simulink model "sstv_receive"  (R2022a)
settings: Solver=FixedStepAuto  StartTime=0.0  StopTime=inf  FixedStep=0.1  RelTol=1e-3
model workspace (MAT data in the model file):
  fc = 1900
  fs = 48000
  lowpassCoefficients = [1.94546975214e-19 0.000106803508505 0.000221855618981 0.000348475799787 0.000488506591805 0.000641464389411 0.000803832818304 0.000968577760455 0.00112495129873 0.00125863449656 0.00135224694036 0.0013862256488 0.0013400488594 0.00119375308299 0.000929666484831 0.000534259876887 -7.53869528953e-19 -0.000672920321007 -0.0014751031701 -0.00238684026913 -0.00337749050162 -0.004405428105 -0.00541862150018 -0.00635586948879 -0.00714868473972 -0.00772377615627 -0.00800604407884 -0.00792196758844 -0.00740323359218 -0.00639043482282 -0.00483664995141 -0.00271071482507 1.87251463643e-18 0.00328747373601 0.00712172383887 0.0114504055026 0.0161993872459 0.0212743208351 0.0265631745006 0.031939649272 0.0372673519447 0.0424045572336 0.0472093583951 0.0515449818895 0.0552850289624 0.0583184061493 0.0605537178776 0.0619229170777 0.0623840429476 0.0619229170777 0.0605537178776 0.0583184061493 0.0552850289624 0.0515449818895 0.0472093583951 0.0424045572336 0.0372673519447 0.031939649272 0.0265631745006 0.0212743208351 0.0161993872459 0.0114504055026 0.00712172383887 0.00328747373601 1.87251463643e-18 -0.00271071482507 -0.00483664995141 -0.00639043482282 -0.00740323359218 -0.00792196758844 -0.00800604407884 -0.00772377615627 -0.00714868473972 -0.00635586948879 -0.00541862150018 -0.004405428105 -0.00337749050162 -0.00238684026913 -0.0014751031701 -0.000672920321007 -7.53869528953e-19 0.000534259876887 0.000929666484831 0.00119375308299 0.0013400488594 0.0013862256488 0.00135224694036 0.00125863449656 0.00112495129873 0.000968577760455 0.000803832818304 0.000641464389411 0.000488506591805 0.000348475799787 0.000221855618981 0.000106803508505 1.94546975214e-19]
  minimumEnvelope = 1e-05
settings Model: Creator=luoch  LastModifiedBy=luoch
settings OptimizationCC: DefaultParameterBehavior=Inlined  EnhancedBackFolding=on  PassReuseOutputArgsAs=Individual arguments  ZeroExternalMemoryAtStartup=off  ZeroInternalMemoryAtStartup=off  OptimizeBlockOrder=speed  DifferentSizesBufferReuse=on  OptimizationCustomize=off  EfficientTunableParamExpr=on
settings DebuggingCC: ParameterTunabilityLossMsg=error
settings HardwareCC: ProdBitPerLong=64  ProdLargestAtomicInteger=LongLong  ProdLargestAtomicFloat=Double  ProdLongLongMode=on  ProdHWDeviceType=ARM Compatible->ARM Cortex-A (64-bit)
settings ModelReferenceCC: EnableRefExpFcnMdlSchedulingChecks=off
settings SFSimCC: MATLABDynamicMemAlloc=off
settings RTWCC: SystemTargetFile=ert.tlc  GenCodeOnly=on  TemplateMakefile=ert_default_tmf  GPUComputeCapability=5.0
settings CodeAppCC: ForceParamTrailComments=on  IgnoreCustomStorageClasses=off  OperatorAnnotations=on  SimulinkDataObjDesc=on  SFDataObjDesc=on  InsertBlockDesc=on
settings ERTTargetCC: TargetLangStandard=C99 (ISO)  InlinedParameterPlacement=NonHierarchical  RootIOFormat=Part of model data structure  ERTCustomFileTemplate=example_file_process.tlc
settings ConfigComp: CovBoundaryAbsTol=1.0e-5

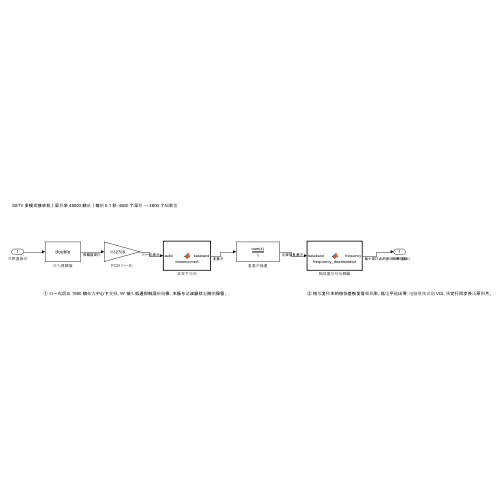
[thumbnail: Simulink's stored preview of the top-level diagram]
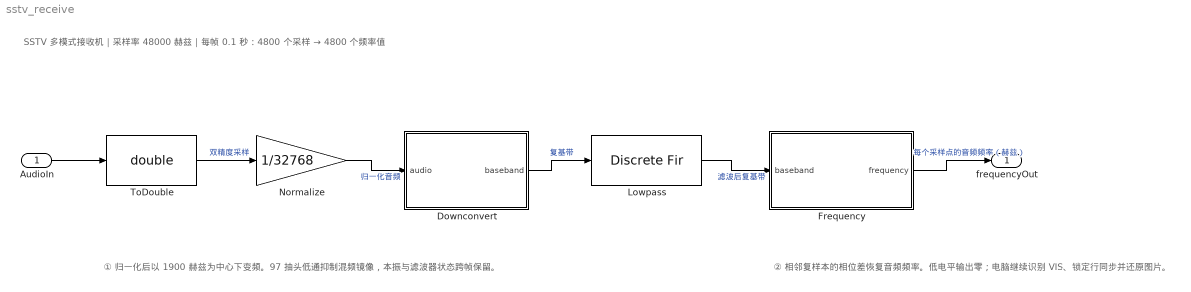
== system sstv_receive ==
  note: SSTV 多模式接收机｜采样率 48000 赫兹｜每帧 0.1 秒：4800 个采样 → 4800 个频率值
  note: ① 归一化后以 1900 赫兹为中心下变频。97 抽头低通抑制混频镜像，本振与滤波器状态跨帧保留。
  note: ② 相邻复样本的相位差恢复音频频率。低电平输出零；电脑继续识别 VIS、锁定行同步并还原图片。
  AudioIn : Inport  OutDataTypeStr=int16  PortDimensions=4800  SampleTime=0.1
      settings: AttributesFormatString=单声道音频
  Downconvert : MATLAB Function  Description=源文件：model/downconvert.m。修改后运行 build_model 更新模型。  TreatAsAtomicUnit=on
      settings: AttributesFormatString=正交下变频
  Frequency : MATLAB Function  Description=源文件：model/frequency_discriminator.m。修改后运行 build_model 更新模型。  TreatAsAtomicUnit=on
      settings: AttributesFormatString=相位差鉴频与静噪
  Lowpass : DiscreteFir  Coefficients=lowpassCoefficients  InputProcessing=Columns as channels (frame based)
      settings: AttributesFormatString=复基带低通
  Normalize : Gain  Gain=1/32768
      settings: AttributesFormatString=PCM 归一化
  ToDouble : DataTypeConversion  OutDataTypeStr=double  SaturateOnIntegerOverflow=off  RndMeth=Floor
      settings: AttributesFormatString=转为双精度
  frequencyOut : Outport
      settings: AttributesFormatString=频率输出
  wires:
  AudioIn/1 -> ToDouble/1
  ToDouble/1 -> Normalize/1  "双精度采样"
  Normalize/1 -> Downconvert/1(audio)  "归一化音频"
  Downconvert/1(baseband) -> Lowpass/1  "复基带"
  Lowpass/1 -> Frequency/1(baseband)  "滤波后复基带"
  Frequency/1(frequency) -> frequencyOut/1  "每个采样点的音频频率（赫兹）"

== matlab function sstv_receive/Frequency ==
  data: baseband input; frequency output; fc parameter; fs parameter; minimumEnvelope parameter
function frequency = frequency_discriminator(baseband,fc, fs, minimumEnvelope)
%#codegen
% 相邻复样本共轭相乘，取相位差得到瞬时频率；低电平以 0 标为不可用。
persistent previous
if isempty(previous),previous=complex(0);end
frequency=zeros(4800,1);
for k=1:4800
    current=baseband(k);
    if abs(current)>=minimumEnvelope && abs(previous)>=minimumEnvelope
        product=current*conj(previous);
        frequency(k)=fc+fs/(2*pi)*atan2(imag(product),real(product));
    end
    previous=current;
end
end

== matlab function sstv_receive/Downconvert ==
  data: audio input; baseband output; fc parameter; fs parameter
function baseband = downconvert(audio,fc, fs)
%#codegen
% 相位连续地把音频移到以 1900 Hz 为中心的复基带，跨帧保存本振相位。
persistent phase
if isempty(phase),phase=0;end
baseband=complex(zeros(4800,1));
for k=1:4800
    baseband(k)=audio(k)*complex(cos(phase),-sin(phase));
    phase=phase+2*pi*fc/fs;
    if phase>=2*pi,phase=phase-2*pi;end
end
end
